simulink model "malha_controle_tempo_continuo"  (R2020b)
settings: Solver=VariableStepAuto  StartTime=0.0  StopTime=10.0  RelTol=1e-3
settings Model: Creator=souza  LastModifiedBy=souza

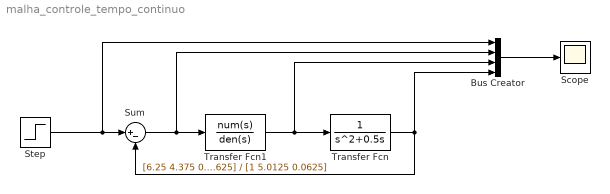
== system malha_controle_tempo_continuo ==
  Bus Creator : BusCreator  Inputs=4
  Scope : Scope
  Step : Step  Time=0  SampleTime=0
  Sum : Sum  Inputs=|+-
  Transfer Fcn : TransferFcn  Denominator=[1 0.5 0]
  Transfer Fcn1 : TransferFcn  Numerator=[6.25 4.375 0.625]  Denominator=[1 5.0125 0.0625]
  wires:
  Bus Creator/1 -> Scope/1
  Step/1 -> Bus Creator/1, Sum/1
  Sum/1 -> Bus Creator/2, Transfer Fcn1/1
  Transfer Fcn1/1 -> Bus Creator/3, Transfer Fcn/1
  Transfer Fcn/1 -> Sum/2, Bus Creator/4
